simulink model "bl_sat_dpl_fh_freq"  (R2013a)
settings: Solver=ode3  StartTime=0.0  StopTime=1  FixedStep=2  RelTol=1e-3
undefined symbols (not defined in the file or in its folder): magnitude, n, wholesignal
libraries: UndergraduateResearch x3, dspxfrm3 x3, dspstat3 x2, dspmtrx3 x2, dspindex x1, simulink x1
settings Model: Creator=dmiralles  LastModifiedBy=dmiralles

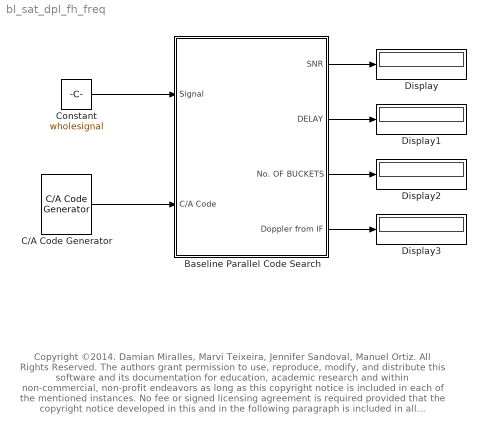
== system bl_sat_dpl_fh_freq ==
  note: Copyright ©2014.  Damian Miralles, Marvi Teixeira, Jennifer Sandoval, Manuel Ortiz. All Rights Reserved.
      | The authors grant permission to use, reproduce, modify, and distribute this software and its documentation for
      | education,  academic research and within non-commercial, non-profit endeavors as long as this copyright notice
      |  is included in each of the mentioned instances. No fee or signed licensing agreement is required provided that
      | the copyright notice developed in this and in the following  paragraph is included in all reproductions,  alterations,
      | and distributions of the software or its  documentation. Contact the authors regarding any commercial licensing needs.
      |
      | THIS EXPERIMENTAL SOFTWARE AND RELATED DOCUMENTATION ARE PROVIDED “AS IS” AND
      |  NO, EXPLICIT OR IMPLICT, CLAIMS REGARDING THEIR ACCURACY OR SUITABILITY ARE MADE.
      | USERS ARE RESPONSIBLE FOR SOFTWARE VALIDATION REGARDING THEIR PARTICULAR
      |  APPLICATION. NO UPDATES WILL BE OFFERED. VERY LIMITED SUPPORT COULD BE PROVIDED,
      |  BUT NOT GUARANTEED, ON A CASE BY CASE BASIS, DEPENDING ON THE AVAILABLE TIME
      |  RESOURCES AT THE TIME OF THE REQUEST.
      | (dmiralles2009@gmail.com,  cc: mteixeir@ieee.org )
  Baseline Parallel Code Search : Subsystem  TreatAsAtomicUnit=on  mask{ssize=763840, ifreq=9548000, fs=38192000, satellite=22, threshold=10}
      mask prompts: ssize "Signal Size in Samples"; ifreq "Intermediate Frequency(Hz)"; fs "Sampling Frequency(Hz)"; satellite "Desired Satellite PRN"
      mask help:
      | The block implements the Parallel Code Search Acquisition method of a real time raw GPS signal. The block receives two input parameters, where signal is the raw gps signal and C/A code is the local generated code used as a method of comparison.
      | The block has several parameters to achieve its final functionality, the Signal Size is the size of the signal in samples that would be passed to the code, this value have to be an integer multiple of (sampling frequency/1000).
      | The intermediate frequency, expressed in Hertz , is the frequency to which the carrier frequency is shifted as an intermediate step in transmission or reception.
      | The sampling frequency defines the number of samples per unit of time (usually seconds) taken from a continuous signal to make a discrete signal.
      | The Desireed Satellite parameter defines the satellite that the user whcih to target in the simulation process if it is expected to be on the raw signal.
  C/A Code Generator : UndergraduateResearch/C//A Code Generator  fs=38192000  sat=22
  Constant : Constant  Value=wholesignal
  Display{,1..3} (4 alike) : Display
  wires:
  Constant/1 -> Baseline Parallel Code Search/1(Signal)
  C/A Code Generator/1 -> Baseline Parallel Code Search/2(C/A Code)
  Baseline Parallel Code Search/1(SNR) -> Display/1
  Baseline Parallel Code Search/2(DELAY) -> Display1/1
  Baseline Parallel Code Search/3(No. OF BUCKETS) -> Display2/1
  Baseline Parallel Code Search/4(Doppler from IF) -> Display3/1

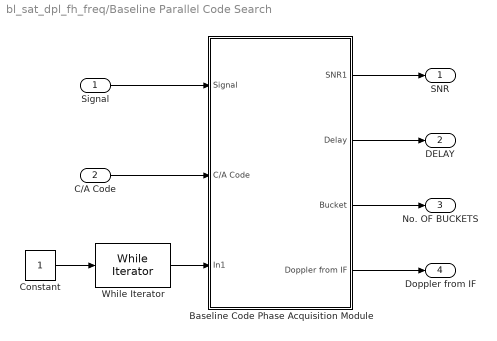
== system bl_sat_dpl_fh_freq/Baseline Parallel Code Search ==
  Signal : Inport
  C/A Code : Inport  Port=2
  Baseline Code Phase Acquisition Module : Subsystem  TreatAsAtomicUnit=on  mask{fs=fs}
      mask prompts: fs "Sampling Frequency"
  Constant : Constant
  While Iterator : WhileIterator  MaxIters=21  WhileBlockType=do-while  ResetStates=reset  ShowIterationPort=on
  SNR : Outport
  DELAY : Outport  Port=2
  No. OF BUCKETS : Outport  Port=3
  Doppler from IF : Outport  Port=4
  wires:
  Baseline Code Phase Acquisition Module/1(SNR1) -> SNR/1
  Baseline Code Phase Acquisition Module/2(Delay) -> DELAY/1
  Baseline Code Phase Acquisition Module/3(Bucket) -> No. OF BUCKETS/1
  While Iterator/1 -> Baseline Code Phase Acquisition Module/3(In1)
  Baseline Code Phase Acquisition Module/4(Doppler from IF) -> Doppler from IF/1
  C/A Code/1 -> Baseline Code Phase Acquisition Module/2(C/A Code)
  Signal/1 -> Baseline Code Phase Acquisition Module/1(Signal)
  Constant/1 -> While Iterator/1

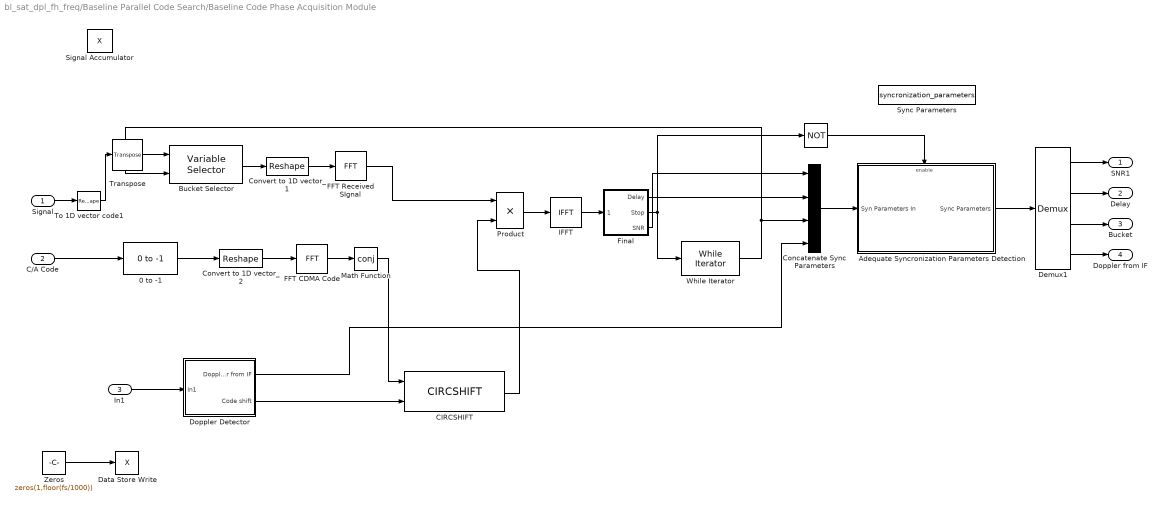
== system bl_sat_dpl_fh_freq/Baseline Parallel Code Search/Baseline Code Phase Acquisition Module ==
  Signal : Inport
  C/A Code : Inport  Port=2
  In1 : Inport  Port=3
  " " : Logic  Operator=NOT  AllPortsSameDT=off  OutDataTypeStr=boolean
  " 0 to -1" : UndergraduateResearch/ 0 to -1
  Adequate Syncronization Parameters Detection : Subsystem  TreatAsAtomicUnit=on
  Bucket Selector : dspindex/Variable Selector  NumInputs=1  rowsOrCols=Rows  IdxMode=Variable  Elements=[1 3]  ZerOneIdxMode=One-based  errmode=Clip Index  FillMode=off  FillValues=0
  CIRCSHIFT : UndergraduateResearch/CIRCSHIFT
  Concatenate Sync Parameters : Concatenate  NumInputs=4
  Convert to 1D vector_1 : Reshape  OutputDimensions=[1023,40]
  Convert to 1D vector_2 : Reshape  OutputDimensions=[1023,40]
  Data Store Write : DataStoreWrite  DataStoreName=X
  Demux1 : Demux
  Doppler Detector : Subsystem
  FFT CDMA Code : dspxfrm3/FFT  CompMethod=Table lookup  TableOpt=NEW  TableOptActive=Speed  BitRevOrder=off  InheritFFTLength=on  FFTLength=1024  RowConvenienceOn=on  FFTImplementation=FFTW  SkipNorm=off  firstCoeffDataTypeStr=Inherit: Same word length as input  firstCoeffLastDataTypeStr=Inherit: Same word length as input  outputMin=[]  outputMax=[]  roundingMode=Floor  overflowMode=off
  FFT Received SIgnal : dspxfrm3/FFT  CompMethod=Table lookup  TableOpt=NEW  TableOptActive=Speed  BitRevOrder=off  InheritFFTLength=on  FFTLength=1024  RowConvenienceOn=on  FFTImplementation=FFTW  SkipNorm=off  firstCoeffDataTypeStr=Inherit: Same word length as input  firstCoeffLastDataTypeStr=Inherit: Same word length as input  outputMin=[]  outputMax=[]  roundingMode=Floor  overflowMode=off
  Final : Subsystem
      mask help: The Final block receives an IFFT and returns if the SNR passed the threshhold and also outputs the SNR and the delay. It uses a variable to accumulate the signal adds it to IFFT and stores it. It detects the maximum value in the signal with the index and assings a 0 to remove the peak to be able to calculate the mean and obtain the SNR.
  IFFT : dspxfrm3/IFFT  CompMethod=Table lookup  TableOpt=NEW  TableOptActive=Speed  BitRevOrder=off  cs_in=off  SkipNorm=on  InheritFFTLength=on  FFTLength=1024  mode=Complex  outSamplingMode=Sample based  RowConvenienceOn=on  FFTImplementation=FFTW  firstCoeffDataTypeStr=Inherit: Same word length as input  firstCoeffLastDataTypeStr=Inherit: Same word length as input  outputMin=[]  outputMax=[]  roundingMode=Floor  overflowMode=off
  Math Function : Math  Operator=conj  SaturateOnIntegerOverflow=on
  Product : Product  RndMeth=Zero
  Signal Accumulator : DataStoreMemory  DataStoreName=X  ReadBeforeWriteMsg=warning  WriteAfterWriteMsg=warning  WriteAfterReadMsg=warning  InitialValue=zeros(1,floor(fs/1000))  VectorParams1D=off
  Sync Parameters : DataStoreMemory  DataStoreName=syncronization_parameters  ReadBeforeWriteMsg=warning  WriteAfterWriteMsg=warning  WriteAfterReadMsg=warning  InitialValue=zeros(1,4)
  To 1D vector code1 : Reshape  OutputDimensionality=Customize  OutputDimensions=[(n),ssize/(n)]
  Transpose : dspmtrx3/Transpose  Hermitian=off  overflowFlag=off
  While Iterator : WhileIterator  MaxIters=10  WhileBlockType=do-while  ResetStates=reset  ShowIterationPort=on  OutputDataType=double
  Zeros : Constant  Value=zeros(1,floor(fs/1000))
  SNR1 : Outport
  Delay : Outport  Port=2
  Bucket : Outport  Port=3
  Doppler from IF : Outport  Port=4
  wires:
  FFT CDMA Code/1 -> Math Function/1
  FFT Received SIgnal/1 -> Product/1
  Product/1 -> IFFT/1
  IFFT/1 -> Final/1(" ")
  Convert to 1D vector_2/1 -> FFT CDMA Code/1
  C/A Code/1 -> " 0 to -1"/1
  " 0 to -1"/1 -> Convert to 1D vector_2/1
  In1/1 -> Doppler Detector/1(In1)
  Math Function/1 -> CIRCSHIFT/1
  CIRCSHIFT/1 -> Product/2
  Doppler Detector/2(Code shift) -> CIRCSHIFT/2
  Bucket Selector/1 -> Convert to 1D vector_1/1
  Convert to 1D vector_1/1 -> FFT Received SIgnal/1
  Zeros/1 -> Data Store Write/1
  Doppler Detector/1(Doppler from IF) -> Concatenate Sync Parameters/4
  Final/3("SNR ") -> Concatenate Sync Parameters/1
  Final/1(Delay) -> Concatenate Sync Parameters/2
  While Iterator/1 -> Bucket Selector/2, Concatenate Sync Parameters/3
  Concatenate Sync Parameters/1 -> Adequate Syncronization Parameters Detection/1(Syn Parameters In)
  Adequate Syncronization Parameters Detection/1("Sync Parameters ") -> Demux1/1
  Final/2(Stop) -> " "/1, While Iterator/1
  Demux1/1 -> SNR1/1
  Demux1/2 -> Delay/1
  Demux1/3 -> Bucket/1
  Demux1/4 -> Doppler from IF/1
  " "/1 -> Adequate Syncronization Parameters Detection/Enable
  Signal/1 -> To 1D vector code1/1
  To 1D vector code1/1 -> Transpose/1
  Transpose/1 -> Bucket Selector/1

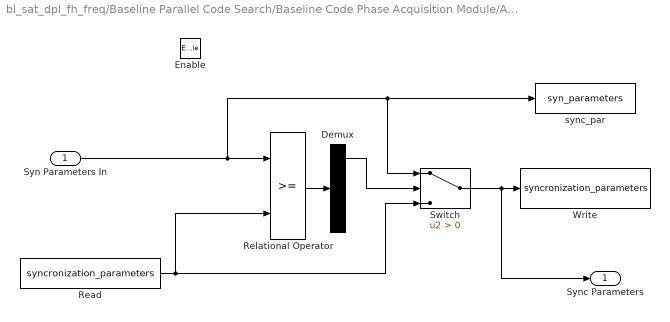
== system bl_sat_dpl_fh_freq/Baseline Parallel Code Search/Baseline Code Phase Acquisition Module/Adequate Syncronization Parameters Detection ==
  Syn Parameters In : Inport
  Enable : EnablePort  StatesWhenEnabling=reset
  Demux : Demux
  Read : DataStoreRead  DataStoreName=syncronization_parameters
  Relational Operator : RelationalOperator  OutDataTypeStr=boolean
  Switch : Switch  Criteria=u2 > Threshold
  Write : DataStoreWrite  DataStoreName=syncronization_parameters
  sync_par : ToWorkspace  VariableName=syn_parameters  SampleTime=-1
  "Sync Parameters " : Outport
  wires:
  Read/1 -> Switch/3, Relational Operator/2
  Switch/1 -> "Sync Parameters "/1, Write/1
  Syn Parameters In/1 -> Relational Operator/1, sync_par/1, Switch/1
  Relational Operator/1 -> Demux/1
  Demux/1 -> Switch/2

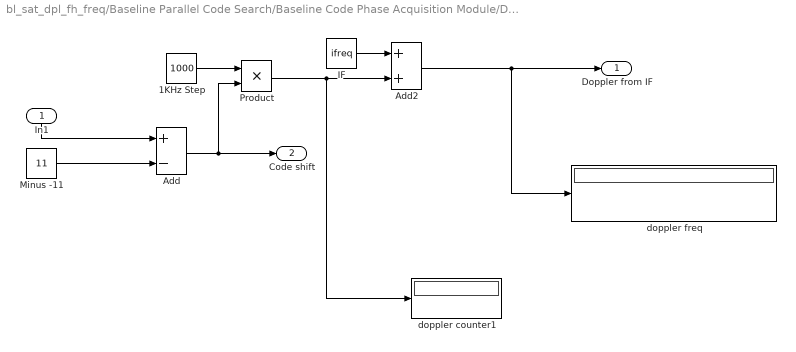
== system bl_sat_dpl_fh_freq/Baseline Parallel Code Search/Baseline Code Phase Acquisition Module/Doppler Detector ==
  In1 : Inport
  1KHz Step : Constant  Value=1000
  Add : Sum  Inputs=+-
  Add2 : Sum
  IF : Constant  Value=ifreq
  Minus -11 : Constant  Value=11
  Product : Product
  doppler counter1 : Display
  doppler freq : Display
  Doppler from IF : Outport
  Code shift : Outport  Port=2
  wires:
  Product/1 -> Add2/2, doppler counter1/1
  1KHz Step/1 -> Product/1
  Add2/1 -> doppler freq/1, Doppler from IF/1
  IF/1 -> Add2/1
  Minus -11/1 -> Add/2
  In1/1 -> Add/1
  Add/1 -> Code shift/1, Product/2

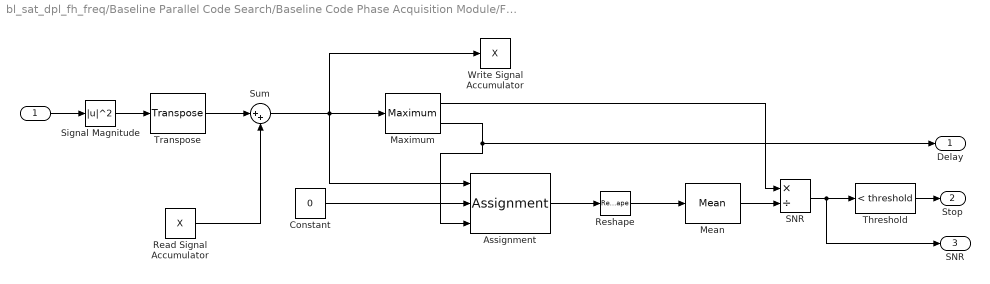
== system bl_sat_dpl_fh_freq/Baseline Parallel Code Search/Baseline Code Phase Acquisition Module/Final ==
  " " : Inport
  " Read Signal Accumulator" : DataStoreRead  DataStoreName=X
  Assignment : Assignment  IndexOptions=Index vector (port)  Indices=1  OutputSizes=1
  Constant : Constant  Value=0
  Maximum : dspstat3/Maximum  fcn=Value and Index  reset=None  InputProcessing=Columns as channels (frame based)  indexBase=One  operateOver=Each column  Dimension=1  colComp=on  operation=maximum  roiEnable=off  roiType=Rectangles  roiPortion=Entire ROI  roiOutput=Individual statistics for each ROI  roiFlag=off  accumDataTypeStr=Inherit: Same as product output  accumLastDataTypeStr=Inherit: Same as product output  roundingMode=Floor  overflowMode=off
  Mean : dspstat3/Mean  run=off  reset_popup=None  InputProcessing=Columns as channels (frame based)  directionMode=Entire input  dimension=1  treatSBRowAsCol=on  roiEnable=off  roiType=Rectangles  roiPortion=Entire ROI  roiOutput=Individual statistics for each ROI  roiFlag=off  outputDataTypeStr=Inherit: Same as accumulator  outputLastDataTypeStr=Inherit: Same as accumulator  outputMin=[]  outputMax=[]  roundingMode=Floor  overflowMode=off
  Reshape : Reshape
  SNR : Product  Inputs=*/
  Signal Magnitude : Math  Operator=magnitude^2  SaturateOnIntegerOverflow=on
  Sum : Sum  Inputs=|++
  Threshold : simulink/Logic and Bit Operations/Compare To Constant  relop=<  const=threshold  OutDataTypeStr=boolean
  Transpose : dspmtrx3/Transpose  Hermitian=off  overflowFlag=off
  Write Signal Accumulator : DataStoreWrite  DataStoreName=X
  Delay : Outport
  Stop : Outport  Port=2
  "SNR " : Outport  Port=3
  wires:
  Threshold/1 -> Stop/1
  Mean/1 -> SNR/2
  SNR/1 -> Threshold/1, "SNR "/1
  Reshape/1 -> Mean/1
  Maximum/1 -> SNR/1
  Sum/1 -> Write Signal Accumulator/1, Assignment/1, Maximum/1
  " Read Signal Accumulator"/1 -> Sum/2
  " "/1 -> Signal Magnitude/1
  Transpose/1 -> Sum/1
  Signal Magnitude/1 -> Transpose/1
  Assignment/1 -> Reshape/1
  Constant/1 -> Assignment/2
  Maximum/2 -> Delay/1, Assignment/3
